simulink model "EKF_model"  (R2024b)
settings: Solver=VariableStepAuto  StartTime=0.0  StopTime=0.2  FixedStep=2e-7  RelTol=1e-3
InitFcn:
  | pn = 4;
  | Ld = 8.5e-3;
  | Lq = 8.5e-3;
  | Ls = Ld;
  | R = 2.875;
  | phi = 0.175;
  | J = 0.001;
  | B = 0.000;
undefined symbols (not defined in the file or in its folder): DiscIntNeverNeededParam
libraries: spsGroundLib x1, spsUniversalBridgeLib x1, spsPermanentMagnetSynchronousMachineLib x1, spsSVPWMGenerator2LevelLib x1, spsDCVoltageSourceLib x1, spspowerguiLib x1

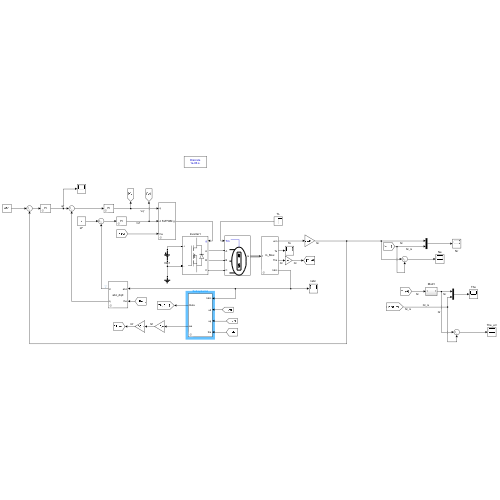
[thumbnail: Simulink's stored preview of the top-level diagram]
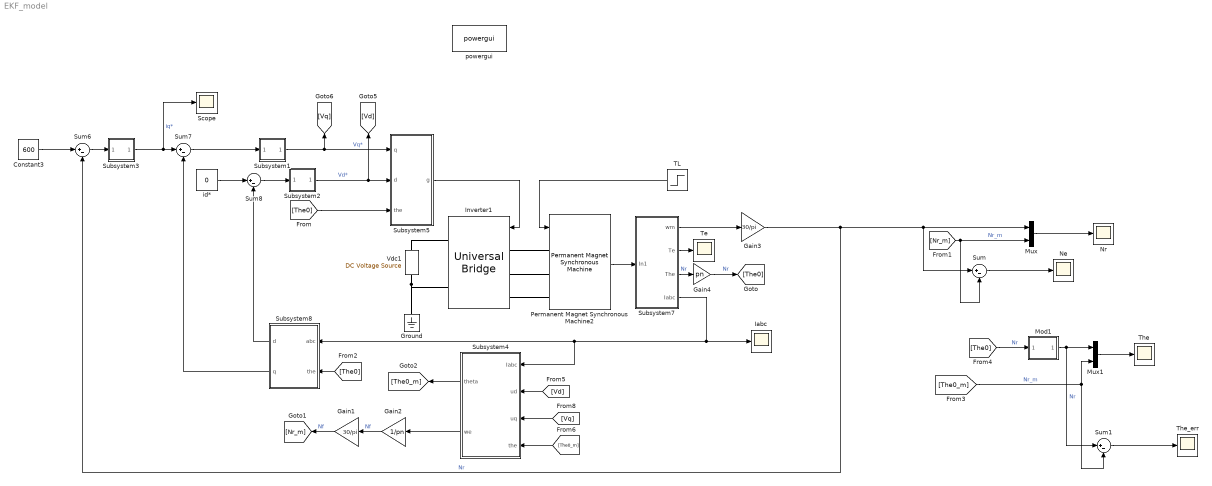
== system EKF_model ==
  Constant3 : Constant  Value=600
  Gain1 : Gain  Gain=30/pi
  Gain2 : Gain  Gain=1/pn
  Gain3 : Gain  Gain=30/pi
  Gain4 : Gain  Gain=pn
  Ground : spsGroundLib/Ground  LConnTagsString=a
  Iabc : Scope
  Inverter1 : spsUniversalBridgeLib/Universal Bridge  Arms=3  SnubberResistance=1e5  SnubberCapacitance=inf  Device=MOSFET / Diodes  Ron=1e-3  Lon=0  ForwardVoltages="[  0  0  ]"  ForwardVoltage=0  GTOparameters=[ 10e-6 , 20e-6 ]  IGBTparameters=[ 1e-6 , 2e-6 ]  Measurements=None  Measurements_2=None  converterType=Rectifier
  Mod1 : Subsystem
  Mux : Mux  Inputs=2
  Mux1 : Mux  Inputs=2
  Ne : Scope
  Nr : Scope
  Permanent Magnet Synchronous Machine2 : spsPermanentMagnetSynchronousMachineLib/Permanent Magnet Synchronous Machine  NbPhases=3  FluxDistribution=Sinusoidal  RotorType=Salient-pole  MechanicalLoad=Torque Tm  PresetModel=No  ShowDetailedParameters=on  MeasurementBus=off  Resistance=R  Inductance=8.5e-3  dqInductances=[Ld Lq]  La=0.000395  MachineConstant=Flux linkage established by magnets (V.s)  Flux=phi  VoltageCst=126.966  TorqueCst=1.05  Flat=120  Mechanical=[J B pn 0]  PolePairs=2  InitialConditions=[0,0, 0,0]  InitialConditions5ph=[0 0 0 0 0 0]  RefAngle=Aligned with phase A axis (original Park)  IterativeDiscreteModel=Trapezoidal non iterative  TsBlock=-1  TsPowergui=0
  Scope : Scope
  Subsystem1 : Subsystem  mask{Ki=5000*R, Kp=5000*Lq, int_limit=[-161,161], out_limit=[-161,161], Ts=1/(10e3)}
      mask prompts: Ki "Ki : Integral"; Kp "Kp : Propotional"; int_limit "integral limit : [min, max]"; out_limit "output limit : [min, max]"; Ts "Ts : sample time"
  Subsystem2 : Subsystem  mask{Ki=5000*R, Kp=5000*Ld, int_limit=[-161,161], out_limit=[-161,161], Ts=1/(10e3)}
      mask prompts: Ki "Ki : Integral"; Kp "Kp : Propotional"; int_limit "integral limit : [min, max]"; out_limit "output limit : [min, max]"; Ts "Ts : sample time"
  Subsystem3 : Subsystem  mask{Ki=20, Kp=0.15, int_limit=[-30,30], out_limit=[-30,30], Ts=1/(5e3)}
      mask prompts: Ki "Ki : Integral"; Kp "Kp : Propotional"; int_limit "integral limit : [min, max]"; out_limit "output limit : [min, max]"; Ts "Ts : sample time"
  Subsystem4 : Subsystem  mask{Ts=1/(10e3), wc=300}
      mask prompts: Ts "Ts : sample time"; wc "wc : cross frequency (rad/s)"
  Subsystem5 : Subsystem  mask{Vdc=311}
  Subsystem7 : Subsystem
  Subsystem8 : Subsystem
  Sum{,1,6..8} (5 alike) : Sum  Inputs=|+-
  TL : Step  Time=0.1  After=10  SampleTime=0
  Te : Scope
  The : Scope
  The_err : Scope
  Vdc1 : spsDCVoltageSourceLib/DC Voltage Source  Amplitude=311  Measurements=None
  id* : Constant  Value=0
  powergui : spspowerguiLib/powergui  Priority=1  SimulationMode=Discrete  SampleTime=10e-7  frequency=60  Iterations=50  frequencyindice=0  Pbase=100e6  ErrMax=1e-4  UnitsV=kV  UnitsW=MW  buscounter=0  FunctionMessages=off  echomessages=off  EnableUseOfTLC=off  CurrentSourceSwitches=off  DisableSnubberDevices=off  DisableRonSwitches=off  DisableVfSwitches=off  DisplayEquations=off  AutomaticDiscreteSolvers=off  SolverType=Tustin/Backward Euler (TBE)  Interpol=off  ExternalGateDelay=off  methode=off  Ts=100  x0status=blocks  SPID=on  SwTol=0  HookPort=off  NonlinearTolerance=1e-4  nMaxIteration=100  ContinueOnMaxIteration=off  RestoreLinks=warning  ResistiveCurrentMeasurement=off  Frange=[0:2:500]  Ylog=off  Xlog=on  ShowGrid=off  save=off  variable=ZData  structure=0  ZoomFFT=off  StartTime=0.0  cycles=1  DisplayStyle=1  fundamental=60  FreqAxis=off  MaxFrequency=1000  frequencyindicesteady=1  RmsSteady=1  display=off
  wires:
  Sum7/1 -> Subsystem1/1(Input)
  Sum6/1 -> Subsystem3/1(Input)
  Subsystem3/1(output) -> Scope/1, Sum7/1  "iq*"
  Constant3/1 -> Sum6/1
  Subsystem5/1(g) -> Inverter1/1
  Subsystem7/1(wm) -> Gain3/1
  id*/1 -> Sum8/1
  Subsystem1/1(output) -> [Vq], Subsystem5/1(q)  "Vq*"
  Sum8/1 -> Subsystem2/1(Input)
  Subsystem2/1(output) -> Subsystem5/2(d), [Vd]  "Vd*"
  Subsystem8/2(q) -> Sum7/2
  Subsystem7/2(Te) -> Te/1
  [The0] -> Subsystem5/3(the)
  Gain2/1 -> Gain1/1  "Nf"
  Subsystem4/2(we) -> Gain2/1
  Gain3/1 -> Sum6/2, Sum/1, Mux/1  "Nr"
  Mux/1 -> Nr/1
  Sum/1 -> Ne/1
  Subsystem7/3(The) -> Gain4/1  "Nr"
  TL/1 -> Permanent Magnet Synchronous Machine2/1
  Permanent Magnet Synchronous Machine2/1 -> Subsystem7/1(In1)
  [The0] -> Subsystem8/2(the)
  Gain4/1 -> [The0]  "Nr"
  Gain1/1 -> [Nr_m]  "Nf"
  [Nr_m] -> Sum/2, Mux/2  "Nr_m"
  Subsystem4/1(theta) -> [The0_m]
  [The0] -> Mod1/1(In1)  "Nr"
  Mux1/1 -> The/1
  [The0_m] -> Mux1/2, Sum1/2  "Nr_m"
  Mod1/1(Out1) -> Sum1/1, Mux1/1  "Nr"
  Sum1/1 -> The_err/1
  Subsystem8/1(d) -> Sum8/2
  Subsystem7/4(Iabc) -> Subsystem4/1(Iabc), Subsystem8/1(abc), Iabc/1
  [Vd] -> Subsystem4/2(ud)
  [Vq] -> Subsystem4/3(uq)
  [The0_m] -> Subsystem4/4(the)
  connections:
  Vdc1/LConn1 -- Inverter1/RConn2 -- Ground/LConn1
  Vdc1/RConn1 -- Inverter1/RConn1
  Permanent Magnet Synchronous Machine2/LConn1 -- Inverter1/LConn1
  Inverter1/LConn3 -- Permanent Magnet Synchronous Machine2/LConn3
  Permanent Magnet Synchronous Machine2/LConn2 -- Inverter1/LConn2

== system EKF_model/Mod1 ==
  In1 : Inport
  Constant1 : Constant  Value=2*pi
  Math Function : Math  Operator=mod  SignedPower=on
  Out1 : Outport
  wires:
  In1/1 -> Math Function/1
  Math Function/1 -> Out1/1
  Constant1/1 -> Math Function/2

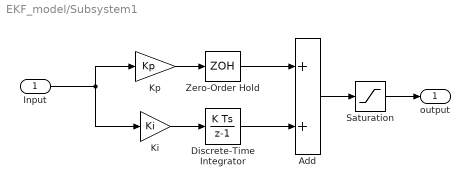
== system EKF_model/Subsystem1 ==
  Input : Inport
  Add : Sum
  Discrete-Time Integrator : DiscreteIntegrator  SampleTime=Ts  LimitOutput=on  UpperSaturationLimit=int_limit(2)  LowerSaturationLimit=int_limit(1)  ICPrevOutput=DiscIntNeverNeededParam  ICPrevScaledInput=DiscIntNeverNeededParam
  Ki : Gain  Gain=Ki
  Kp : Gain  Gain=Kp
  Saturation : Saturate  UpperLimit=out_limit(2)  LowerLimit=out_limit(1)
  Zero-Order Hold : ZeroOrderHold  SampleTime=Ts
  output : Outport
  wires:
  Input/1 -> Ki/1, Kp/1
  Ki/1 -> Discrete-Time Integrator/1
  Discrete-Time Integrator/1 -> Add/2
  Add/1 -> Saturation/1
  Saturation/1 -> output/1
  Kp/1 -> Zero-Order Hold/1
  Zero-Order Hold/1 -> Add/1

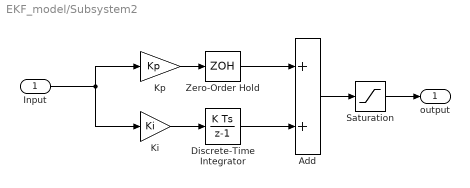
== system EKF_model/Subsystem2 ==
  Input : Inport
  Add : Sum
  Discrete-Time Integrator : DiscreteIntegrator  SampleTime=Ts  LimitOutput=on  UpperSaturationLimit=int_limit(2)  LowerSaturationLimit=int_limit(1)  ICPrevOutput=DiscIntNeverNeededParam  ICPrevScaledInput=DiscIntNeverNeededParam
  Ki : Gain  Gain=Ki
  Kp : Gain  Gain=Kp
  Saturation : Saturate  UpperLimit=out_limit(2)  LowerLimit=out_limit(1)
  Zero-Order Hold : ZeroOrderHold  SampleTime=Ts
  output : Outport
  wires:
  Input/1 -> Ki/1, Kp/1
  Ki/1 -> Discrete-Time Integrator/1
  Discrete-Time Integrator/1 -> Add/2
  Add/1 -> Saturation/1
  Saturation/1 -> output/1
  Kp/1 -> Zero-Order Hold/1
  Zero-Order Hold/1 -> Add/1

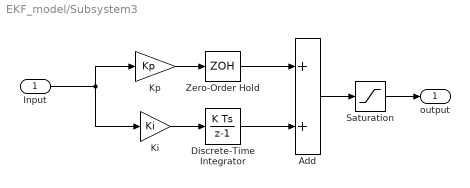
== system EKF_model/Subsystem3 ==
  Input : Inport
  Add : Sum
  Discrete-Time Integrator : DiscreteIntegrator  SampleTime=Ts  LimitOutput=on  UpperSaturationLimit=int_limit(2)  LowerSaturationLimit=int_limit(1)  ICPrevOutput=DiscIntNeverNeededParam  ICPrevScaledInput=DiscIntNeverNeededParam
  Ki : Gain  Gain=Ki
  Kp : Gain  Gain=Kp
  Saturation : Saturate  UpperLimit=out_limit(2)  LowerLimit=out_limit(1)
  Zero-Order Hold : ZeroOrderHold  SampleTime=Ts
  output : Outport
  wires:
  Input/1 -> Ki/1, Kp/1
  Ki/1 -> Discrete-Time Integrator/1
  Discrete-Time Integrator/1 -> Add/2
  Add/1 -> Saturation/1
  Saturation/1 -> output/1
  Kp/1 -> Zero-Order Hold/1
  Zero-Order Hold/1 -> Add/1

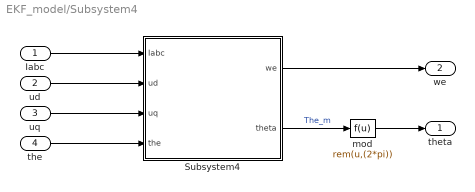
== system EKF_model/Subsystem4 ==
  Iabc : Inport
  ud : Inport  Port=2
  uq : Inport  Port=3
  the : Inport  Port=4
  Subsystem4 : Subsystem
  mod : Fcn  Expr=rem(u,(2*pi))
  theta : Outport
  we : Outport  Port=2
  wires:
  Subsystem4/1(we) -> we/1
  Iabc/1 -> Subsystem4/1(Iabc)
  ud/1 -> Subsystem4/2(ud)
  uq/1 -> Subsystem4/3(uq)
  Subsystem4/2(theta) -> mod/1  "The_m"
  mod/1 -> theta/1
  the/1 -> Subsystem4/4(the)

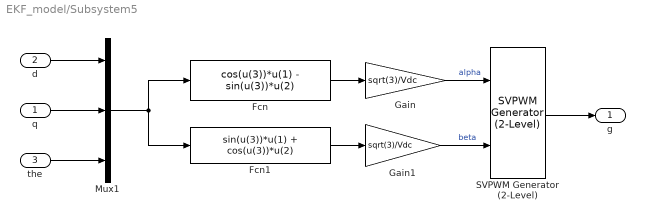
== system EKF_model/Subsystem5 ==
  q : Inport
  d : Inport  Port=2
  the : Inport  Port=3
  Fcn : Fcn  Expr=cos(u(3))*u(1) - sin(u(3))*u(2)
  Fcn1 : Fcn  Expr=sin(u(3))*u(1) + cos(u(3))*u(2)
  Gain : Gain  Gain=sqrt(3)/Vdc
  Gain1 : Gain  Gain=sqrt(3)/Vdc
  Mux1 : Mux  Inputs=3
  SVPWM Generator (2-Level) : spsSVPWMGenerator2LevelLib/SVPWM Generator (2-Level)  InputType=alpha-beta components  SwitchingPattern=Pattern #1  Fc=10e3  ParUref=[0.8 -30 50]  Ts=0
  g : Outport
  wires:
  q/1 -> Mux1/2
  Fcn/1 -> Gain/1
  d/1 -> Mux1/1
  Fcn1/1 -> Gain1/1
  SVPWM Generator (2-Level)/1 -> g/1
  Mux1/1 -> Fcn/1, Fcn1/1
  the/1 -> Mux1/3
  Gain/1 -> SVPWM Generator (2-Level)/1  "alpha"
  Gain1/1 -> SVPWM Generator (2-Level)/2  "beta"

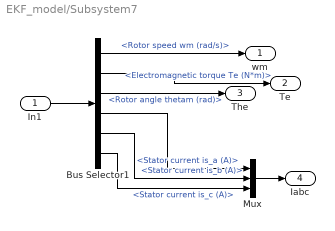
== system EKF_model/Subsystem7 ==
  In1 : Inport
  Bus Selector1 : BusSelector  OutputSignals=Rotor speed wm (rad/s),Electromagnetic torque Te (N*m),Rotor angle thetam (rad),Stator current is_a (A),Stator current is_b (A),Stator current is_c (A)
  Mux : Mux  Inputs=3
  wm : Outport
  Te : Outport  Port=2
  The : Outport  Port=3
  Iabc : Outport  Port=4
  wires:
  In1/1 -> Bus Selector1/1
  Bus Selector1/1 -> wm/1  "<Rotor speed wm (rad/s)>"
  Bus Selector1/2 -> Te/1  "<Electromagnetic torque Te (N*m)>"
  Bus Selector1/3 -> The/1  "<Rotor angle thetam (rad)>"
  Bus Selector1/4 -> Mux/1  "<Stator current is_a (A)>"
  Bus Selector1/5 -> Mux/2  "<Stator current is_b (A)>"
  Bus Selector1/6 -> Mux/3  "<Stator current is_c (A)>"
  Mux/1 -> Iabc/1

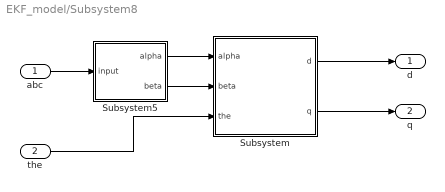
== system EKF_model/Subsystem8 ==
  abc : Inport
  the : Inport  Port=2
  Subsystem : Subsystem
  Subsystem5 : Subsystem
  d : Outport
  q : Outport  Port=2
  wires:
  Subsystem/1(d) -> d/1
  the/1 -> Subsystem/3(the)
  Subsystem5/2(beta) -> Subsystem/2(beta)
  Subsystem5/1(alpha) -> Subsystem/1(alpha)
  abc/1 -> Subsystem5/1(input)
  Subsystem/2(q) -> q/1

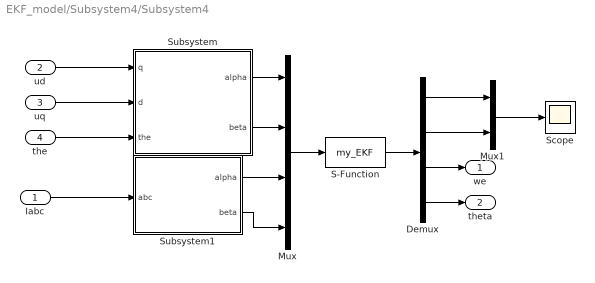
== system EKF_model/Subsystem4/Subsystem4 ==
  Iabc : Inport
  ud : Inport  Port=2
  uq : Inport  Port=3
  the : Inport  Port=4
  Demux : Demux
  Mux : Mux
  Mux1 : Mux  Inputs=2
  S-Function : S-Function  FunctionName=my_EKF  SFunctionDeploymentMode=off  EnableBusSupport=off
  Scope : Scope
  Subsystem : Subsystem
  Subsystem1 : Subsystem
  we : Outport
  theta : Outport  Port=2
  wires:
  ud/1 -> Subsystem/1(q)
  uq/1 -> Subsystem/2(d)
  the/1 -> Subsystem/3(the)
  Iabc/1 -> Subsystem1/1(abc)
  Mux/1 -> S-Function/1
  S-Function/1 -> Demux/1
  Demux/2 -> Mux1/2
  Demux/3 -> we/1
  Demux/4 -> theta/1
  Demux/1 -> Mux1/1
  Mux1/1 -> Scope/1
  Subsystem/2(beta) -> Mux/2
  Subsystem/1(alpha) -> Mux/1
  Subsystem1/1(alpha) -> Mux/3
  Subsystem1/2(beta) -> Mux/4

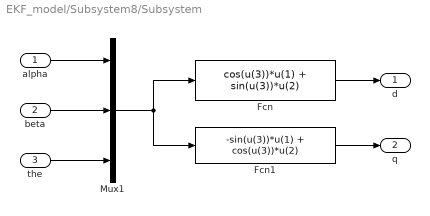
== system EKF_model/Subsystem8/Subsystem ==
  alpha : Inport
  beta : Inport  Port=2
  the : Inport  Port=3
  Fcn : Fcn  Expr=cos(u(3))*u(1) + sin(u(3))*u(2)
  Fcn1 : Fcn  Expr=-sin(u(3))*u(1) + cos(u(3))*u(2)
  Mux1 : Mux  Inputs=3
  d : Outport
  q : Outport  Port=2
  wires:
  Fcn/1 -> d/1
  Mux1/1 -> Fcn/1, Fcn1/1
  the/1 -> Mux1/3
  beta/1 -> Mux1/2
  Fcn1/1 -> q/1
  alpha/1 -> Mux1/1

== system EKF_model/Subsystem8/Subsystem5 ==
  input : Inport
  Demux : Demux  Outputs=3
  Subsystem : Subsystem
  alpha : Outport
  beta : Outport  Port=2
  wires:
  input/1 -> Demux/1
  Demux/1 -> Subsystem/1(a)
  Demux/2 -> Subsystem/2(b)
  Demux/3 -> Subsystem/3(c)
  Subsystem/1(alpha) -> alpha/1
  Subsystem/2(beta) -> beta/1

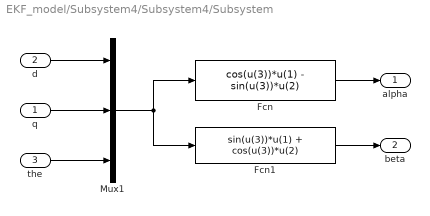
== system EKF_model/Subsystem4/Subsystem4/Subsystem ==
  q : Inport
  d : Inport  Port=2
  the : Inport  Port=3
  Fcn : Fcn  Expr=cos(u(3))*u(1) - sin(u(3))*u(2)
  Fcn1 : Fcn  Expr=sin(u(3))*u(1) + cos(u(3))*u(2)
  Mux1 : Mux  Inputs=3
  alpha : Outport
  beta : Outport  Port=2
  wires:
  Mux1/1 -> Fcn/1, Fcn1/1
  q/1 -> Mux1/2
  the/1 -> Mux1/3
  Fcn/1 -> alpha/1
  Fcn1/1 -> beta/1
  d/1 -> Mux1/1

== system EKF_model/Subsystem4/Subsystem4/Subsystem1 ==
  abc : Inport
  Fcn : Fcn  Expr=2/3*(u(1) - 0.5*u(2) - 0.5*u(3))
  Fcn1 : Fcn  Expr=sqrt(3)/3*(u(2) - u(3))
  alpha : Outport
  beta : Outport  Port=2
  wires:
  Fcn/1 -> alpha/1
  Fcn1/1 -> beta/1
  abc/1 -> Fcn1/1, Fcn/1

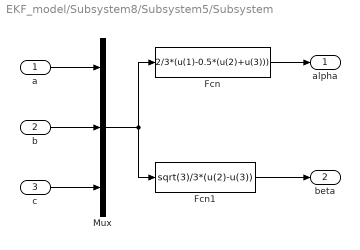
== system EKF_model/Subsystem8/Subsystem5/Subsystem ==
  a : Inport
  b : Inport  Port=2
  c : Inport  Port=3
  Fcn : Fcn  Expr=2/3*(u(1)-0.5*(u(2)+u(3)))
  Fcn1 : Fcn  Expr=sqrt(3)/3*(u(2)-u(3))
  Mux : Mux  Inputs=3
  alpha : Outport
  beta : Outport  Port=2
  wires:
  a/1 -> Mux/1
  b/1 -> Mux/2
  c/1 -> Mux/3
  Mux/1 -> Fcn/1, Fcn1/1
  Fcn/1 -> alpha/1
  Fcn1/1 -> beta/1
